simulink model "lateral_autopilot_2f"  (R2018b)
settings: Solver=VariableStepAuto  StartTime=0.0  StopTime=500  RelTol=1e-3
values from neighbouring files (symbols this model uses):
  A = [ ... (first row only)    [lateral_autopilot_2e_params.m]
  B = [0 0 0 0 7.5]'    [lateral_autopilot_2e_params.m]
  C = [eye(4) zeros(4,1)]    [lateral_autopilot_2e_params.m]
  d = 1.5    [lateral_autopilot_2e_params.m]
  g = 9.81    [lateral_autopilot_2e_params.m]
  kd_phi = (2*zeta_phi*omega_n_phi-a_phi_1)/a_phi_2    [lateral_autopilot_2e_params.m]
  ki_chi = omega_chi_phi^2*vg/g    [lateral_autopilot_2e_params.m]
  kp_chi = 2*zeta_chi*omega_chi_phi*vg/g    [lateral_autopilot_2e_params.m]
  kp_phi = (aileron_max/error_max)*sign(a_phi_2)    [lateral_autopilot_2e_params.m]
  vg = 580*km_h2m_s    (= 161.111111111)    [lateral_autopilot_2e_params.m]
libraries: simulink_extras x3, simulink x1
settings Model: Creator=dino  LastModifiedBy=dino

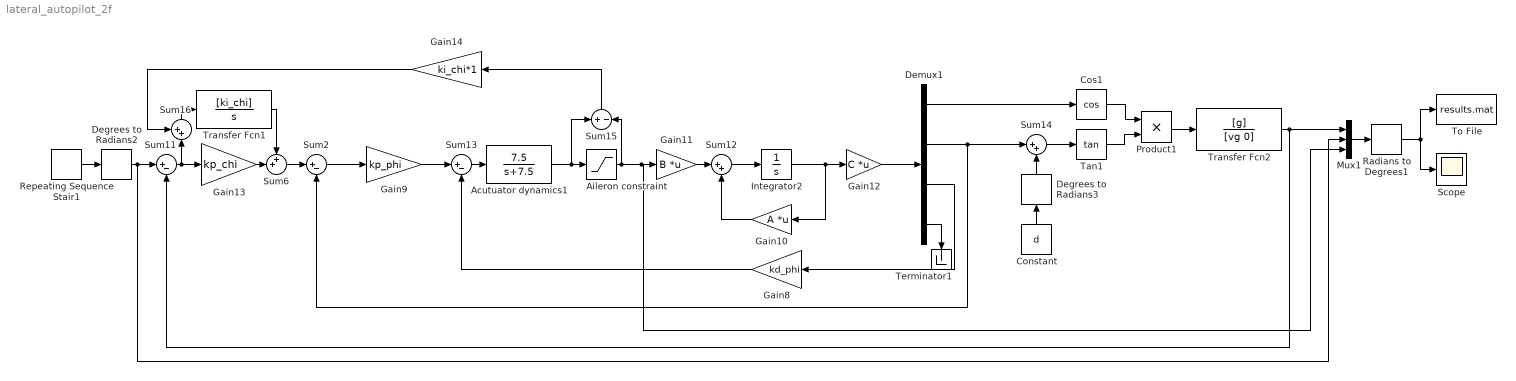
== system lateral_autopilot_2f ==
  Acutuator dynamics1 : TransferFcn  Numerator=[0 7.5]  Denominator=[1 7.5]
  "Aileron constraint " : Saturate  UpperLimit=30*deg2rad  LowerLimit=-30*deg2rad
  Constant : Constant  Value=d
  Cos1 : Trigonometry  Operator=cos
  Degrees to Radians2 : simulink_extras/Transformations/Degrees to Radians
  Degrees to Radians3 : simulink_extras/Transformations/Degrees to Radians
  Demux1 : Demux
  Gain10 : Gain  Gain=A  Multiplication=Matrix(K*u)
  Gain11 : Gain  Gain=B  Multiplication=Matrix(K*u)
  Gain12 : Gain  Gain=C  Multiplication=Matrix(K*u)
  Gain13 : Gain  Gain=kp_chi
  Gain14 : Gain  Gain=ki_chi*1
  Gain8 : Gain  Gain=kd_phi
  Gain9 : Gain  Gain=kp_phi
  Integrator2 : Integrator
  Mux1 : Mux  Inputs=3
  Product1 : Product
  Radians to Degrees1 : simulink_extras/Transformations/Radians to Degrees
  Repeating Sequence Stair1 : simulink/Sources/Repeating Sequence Stair  OutValues=step_series.'  tsamp=60  OutMin=[]  OutMax=[]  OutDataTypeStr=double  OutputDataTypeScalingMode=double  OutDataType=fixdt(0,8)  ConRadixGroup=Best Precision: Vector-wise  OutScaling=2^-12
  Scope : Scope
  Sum11 : Sum  Inputs=|+-
  Sum12 : Sum  Inputs=|++
  Sum13 : Sum  Inputs=|+-
  Sum14 : Sum  Inputs=|++
  Sum15 : Sum  Inputs=+|-
  Sum16 : Sum  Inputs=++|
  Sum2 : Sum  Inputs=|+-
  Sum6 : Sum  Inputs=++|
  Tan1 : Trigonometry  Operator=tan
  Terminator1 : Terminator
  To File : ToFile  Filename=results.mat
  Transfer Fcn1 : TransferFcn  Numerator=[ki_chi]  Denominator=[1 0]
  Transfer Fcn2 : TransferFcn  Numerator=[g]  Denominator=[vg 0]
  wires:
  Demux1/1 -> Cos1/1
  Repeating Sequence Stair1/1 -> Degrees to Radians2/1
  Demux1/4 -> Terminator1/1
  Gain8/1 -> Sum13/2
  Sum14/1 -> Tan1/1
  Cos1/1 -> Product1/1
  Mux1/1 -> Radians to Degrees1/1
  Product1/1 -> Transfer Fcn2/1
  Integrator2/1 -> Gain10/1, Gain12/1
  Sum11/1 -> Sum16/2, Gain13/1
  Gain11/1 -> Sum12/1
  Sum2/1 -> Gain9/1
  Gain13/1 -> Sum6/2
  Gain12/1 -> Demux1/1
  Transfer Fcn1/1 -> Sum6/1
  Sum6/1 -> Sum2/1
  Degrees to Radians2/1 -> Mux1/2, Sum11/1
  Gain9/1 -> Sum13/1
  Transfer Fcn2/1 -> Sum11/2, Mux1/1
  Constant/1 -> Degrees to Radians3/1
  Sum12/1 -> Integrator2/1
  Gain10/1 -> Sum12/2
  Degrees to Radians3/1 -> Sum14/2
  Sum13/1 -> Acutuator dynamics1/1
  Radians to Degrees1/1 -> Scope/1, To File/1
  Tan1/1 -> Product1/2
  Demux1/2 -> Sum2/2, Sum14/1
  Demux1/3 -> Gain8/1
  "Aileron constraint "/1 -> Gain11/1, Mux1/3, Sum15/2
  Acutuator dynamics1/1 -> Sum15/1, "Aileron constraint "/1
  Sum15/1 -> Gain14/1
  Sum16/1 -> Transfer Fcn1/1
  Gain14/1 -> Sum16/1
